simulink model "FIR_Filter"  (R2020b)
settings: Solver=VariableStepAuto  StartTime=0.0  StopTime=10.0  MaxStep=0.002  RelTol=1e-3
settings Model: Creator=ARPITA  LastModifiedBy=ARPITA
settings DataIOCC: SaveOutput=off  SaveTime=off

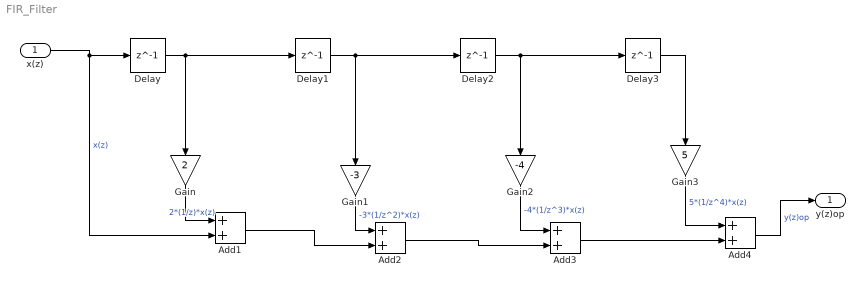
== system FIR_Filter ==
  x(z) : Inport  OutDataTypeStr=double  PortDimensions=1  SampleTime=0
  Add{1..4} (4 alike) : Sum
  Delay{,1..3} (4 alike) : Delay  DelayLength=1
  Gain : Gain  Gain=2
  Gain1 : Gain  Gain=-3
  Gain2 : Gain  Gain=-4
  Gain3 : Gain  Gain=5
  y(z)op : Outport  OutDataTypeStr=double  PortDimensions=1  SampleTime=0
  wires:
  x(z)/1 -> Delay/1, Add1/2  "x(z)"
  Add3/1 -> Add4/2
  Delay/1 -> Gain/1, Delay1/1
  Delay1/1 -> Gain1/1, Delay2/1
  Gain1/1 -> Add2/1  "-3*(1/z^2)*x(z)"
  Add4/1 -> y(z)op/1  "y(z)op"
  Gain2/1 -> Add3/1  "-4*(1/z^3)*x(z)"
  Gain3/1 -> Add4/1  "5*(1/z^4)*x(z)"
  Delay2/1 -> Gain2/1, Delay3/1
  Gain/1 -> Add1/1  "2*(1/z)*x(z)"
  Add2/1 -> Add3/2
  Add1/1 -> Add2/2
  Delay3/1 -> Gain3/1
